simulink model "qdqd_robot"  (R2022b)
settings: Solver=FixedStepAuto  StartTime=0.0  StopTime=10  FixedStep=0.01  RelTol=1e-3  EnableMultiTasking=on
model workspace: external: MATLAB File C:\Users\Tin\Desktop\tailieuhoc\TT Robotics\task2\robot_DataFile2.m (data not in the file)
undefined symbols (not defined in the file): smiData, X, Y, Z
libraries: sm_lib x21, nesl_utility x4, arduinolib x3
settings Model: ExtModeTrigDuration=2  Creator=Tin  LastModifiedBy=Tin
settings OptimizationCC: EnhancedBackFolding=on  PassReuseOutputArgsAs=Individual arguments  ZeroExternalMemoryAtStartup=off  ZeroInternalMemoryAtStartup=off  MaxStackSize=64  OptimizeBlockOrder=speed  DifferentSizesBufferReuse=on  OptimizationCustomize=off  EfficientTunableParamExpr=on
settings DebuggingCC: ParameterTunabilityLossMsg=error
settings HardwareCC: ProdBitPerInt=16  ProdBitPerPointer=16  ProdBitPerSizeT=16  ProdBitPerPtrDiffT=16  ProdLargestAtomicFloat=None  ProdWordSize=8  ProdHWDeviceType=Atmel->AVR
settings SFSimCC: MATLABDynamicMemAlloc=off
settings RTWCC: Description=Embedded Coder  SystemTargetFile=ert.tlc  HardwareBoard=Arduino Uno  TLCOptions=-aInlineSetEventsForThisBaseRateFcn=TLC_FALSE -aSuppressMultiTaskScheduler=TLC_FALSE -aRateBasedStepFcn=1  TemplateMakefile=ert_default_tmf  Toolchain=Arduino AVR  BuildConfiguration=Faster Runs
settings CodeAppCC: ForceParamTrailComments=on  IgnoreCustomStorageClasses=off  OperatorAnnotations=on  SimulinkDataObjDesc=on  SFDataObjDesc=on  InsertBlockDesc=on
settings ERTTargetCC: SupportContinuousTime=on  SupportVariableSizeSignals=on  ExtModeTransport=3  ExtModeStaticAlloc=on  ExtModeAutomaticAllocSize=off  ExtModeStaticAllocSize=250  ExtModeMexFile=ext_xcp  ExtModeIntrfLevel=Level2 - Open

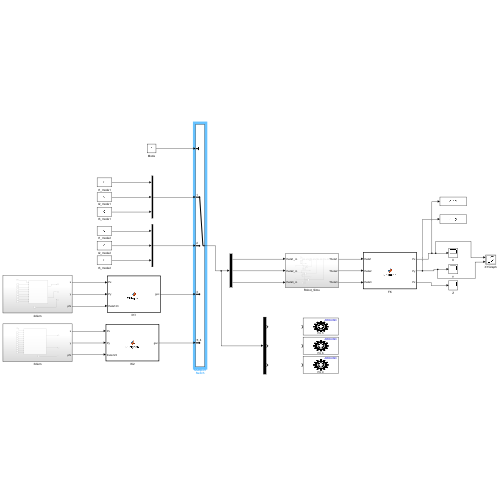
[thumbnail: Simulink's stored preview of the top-level diagram]
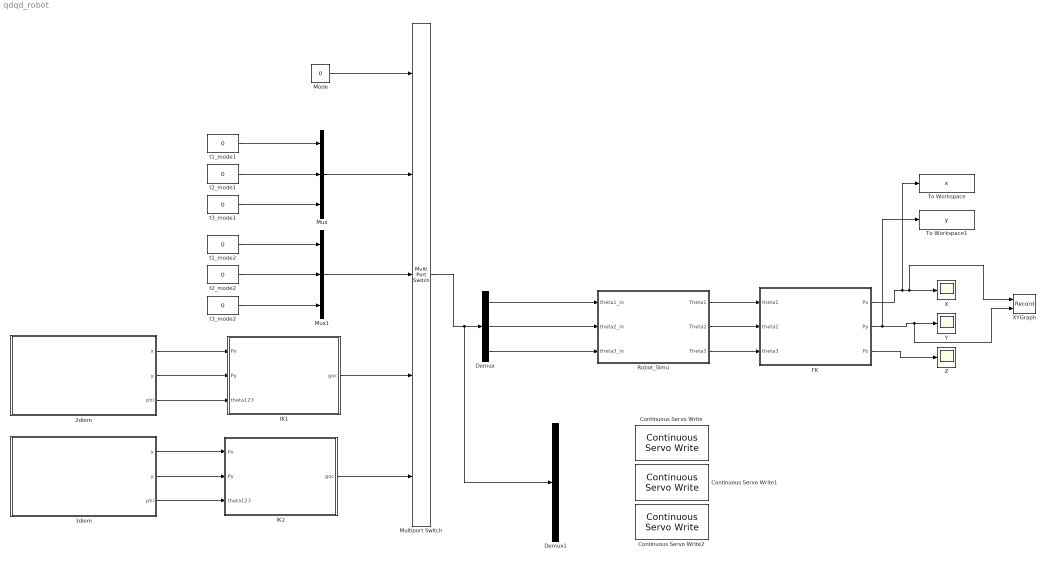
== system qdqd_robot ==
  2diem : Subsystem
  3diem : Subsystem
  Continuous Servo Write : arduinolib/Continuous Servo Write  pinNumber=5  ServoIndex=0  blockPlatform=ARDUINO
  Continuous Servo Write1 : arduinolib/Continuous Servo Write  pinNumber=6  ServoIndex=1  blockPlatform=ARDUINO
  Continuous Servo Write2 : arduinolib/Continuous Servo Write  pinNumber=9  ServoIndex=2  blockPlatform=ARDUINO
  Demux : Demux  Outputs=3
  Demux1 : Demux  Outputs=3
  FK : MATLAB Function  TreatAsAtomicUnit=on
  IK1 : MATLAB Function  TreatAsAtomicUnit=on
  IK2 : MATLAB Function  TreatAsAtomicUnit=on
  Mode : Constant  Value=0
  Multiport Switch : MultiPortSwitch  Inputs=4  DiagnosticForDefault=None  SaturateOnIntegerOverflow=off  InputSameDT=off
  Mux : Mux  Inputs=3
  Mux1 : Mux  Inputs=3
  Robot_Simu : Subsystem
  To Workspace : ToWorkspace  VariableName=x  SampleTime=-1
      settings: Save2DSignal=2-D array (concatenate along first dimension)
  To Workspace1 : ToWorkspace  VariableName=y  SampleTime=-1
      settings: Save2DSignal=2-D array (concatenate along first dimension)
  X : Scope
  XYGraph : Record  FileSettingsInternal="{\"entries\":[{\"content\":{\"excelSettings\":{\"content\":{},\"type\":\"Streamout.ExcelSettings\"}},\"type\":\"Streamout.FileSettingStorage\",\"uuid\":\"e4239a1c-dab3-499a-a52f-9dc0fa17a419\"}],\"packageUris\":[\"http://schema.mathworks.com/mf0/streamout_blocks/R2020a\"],\"version\":\"1.0\"}"  Layout=[1 1]  SignalsInternal="{\"entries\":[{\"content\":{\"signals\":[{\"content\":{\"blockPath\":[\"qdqd_robot/XYGraph\"],\"channel\":[],\"dimensions\":[1],\"domain\":\"qdqd_robot/XYGraph\",\"lineColor\":\"#ff6929\",\"plots\":[],\"port\":1,\"sid\":[\"\"],\"signalID\":171,\"signalName\":\"FK:1\"},\"type\":\"RecordBlkView.Signal\",\"uuid\":\"71b2b6ee-b9d0-4eec-b635-3188d7877590\"},{\"content\":{\"blockPath\":[\"qdqd_robot/XYGraph\"],\"channel\":[],\"dimensions\":[1],\"domain\":\"qdqd_robot/XYGraph\",\"lineColor\":\"#b746ff\",\"plots\":[],\"port\":2,\"sid\":[\"\"],\"signalID\":175,\"signalName\":\"FK:2\"},\"type\":\"RecordBlkView.Signal\",\"uuid\":\"dff031ee-cb77-442e-8ca7-25a6e18e3c29\"}]},\"type\":\"RecordBlkView.InputSignals\",\"uuid\":\"b65a76cf-75d9-49b1-9cf8-3691b3f56b91\"}],\"packageUris\":[\"http://schema.mathworks.com/mf0/streamout_blocks/R2020a\"],\"version\":\"1.0\"}"  VisualizationBindings="{\"xyplotplugin\":{\"info\":[{\"series\":[],\"subplotID\":1}]}}"  CompatibilityTag=XY
  Y : Scope
  Z : Scope
  t1_mode1 : Constant  Value=0
  t1_mode2 : Constant  Value=0
  t2_mode1 : Constant  Value=0
  t2_mode2 : Constant  Value=0
  t3_mode1 : Constant  Value=0
  t3_mode2 : Constant  Value=0
  wires:
  2diem/3(phi) -> IK1/3(theta123)
  2diem/2(y) -> IK1/2(Py)
  3diem/3(phi) -> IK2/3(theta123)
  t2_mode1/1 -> Mux/2
  t3_mode1/1 -> Mux/3
  Mux/1 -> Multiport Switch/2
  Demux/2 -> Robot_Simu/2(theta2_in)
  Demux/3 -> Robot_Simu/3(theta3_in)
  Multiport Switch/1 -> Demux1/1, Demux/1
  t1_mode1/1 -> Mux/1
  3diem/2(y) -> IK2/2(Py)
  3diem/1(x) -> IK2/1(Px)
  Robot_Simu/1(Theta1) -> FK/1(theta1)
  Robot_Simu/2(Theta2) -> FK/2(theta2)
  Robot_Simu/3(Theta3) -> FK/3(theta3)
  FK/1(Px) -> To Workspace/1, XYGraph/1, X/1
  FK/2(Py) -> To Workspace1/1, XYGraph/2, Y/1
  FK/3(Pz) -> Z/1
  Demux/1 -> Robot_Simu/1(theta1_in)
  2diem/1(x) -> IK1/1(Px)
  Mode/1 -> Multiport Switch/1
  IK2/1(goc) -> Multiport Switch/5
  IK1/1(goc) -> Multiport Switch/4
  t1_mode2/1 -> Mux1/1
  Mux1/1 -> Multiport Switch/3
  t3_mode2/1 -> Mux1/3
  t2_mode2/1 -> Mux1/2

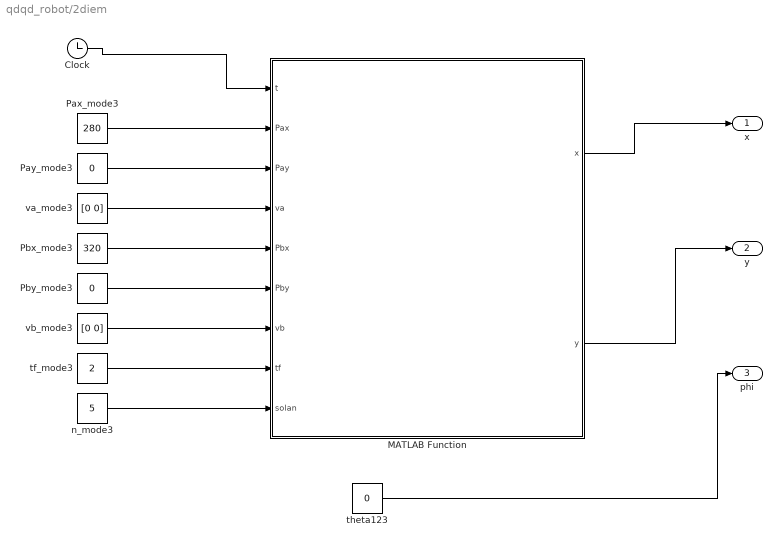
== system qdqd_robot/2diem ==
  Clock : Clock
  MATLAB Function : MATLAB Function  TreatAsAtomicUnit=on
  Pax_mode3 : Constant  Value=280
  Pay_mode3 : Constant  Value=0
  Pbx_mode3 : Constant  Value=320
  Pby_mode3 : Constant  Value=0
  n_mode3 : Constant  Value=5
  tf_mode3 : Constant  Value=2
  theta123 : Constant  Value=0
  va_mode3 : Constant  Value=[0 0]
  vb_mode3 : Constant  Value=[0 0]
  x : Outport
  y : Outport  Port=2
  phi : Outport  Port=3
  wires:
  Pbx_mode3/1 -> MATLAB Function/5(Pbx)
  Pax_mode3/1 -> MATLAB Function/2(Pax)
  Pby_mode3/1 -> MATLAB Function/6(Pby)
  Clock/1 -> MATLAB Function/1(t)
  tf_mode3/1 -> MATLAB Function/8(tf)
  n_mode3/1 -> MATLAB Function/9(solan)
  vb_mode3/1 -> MATLAB Function/7(vb)
  va_mode3/1 -> MATLAB Function/4(va)
  Pay_mode3/1 -> MATLAB Function/3(Pay)
  MATLAB Function/1(x) -> x/1
  theta123/1 -> phi/1
  MATLAB Function/2(y) -> y/1

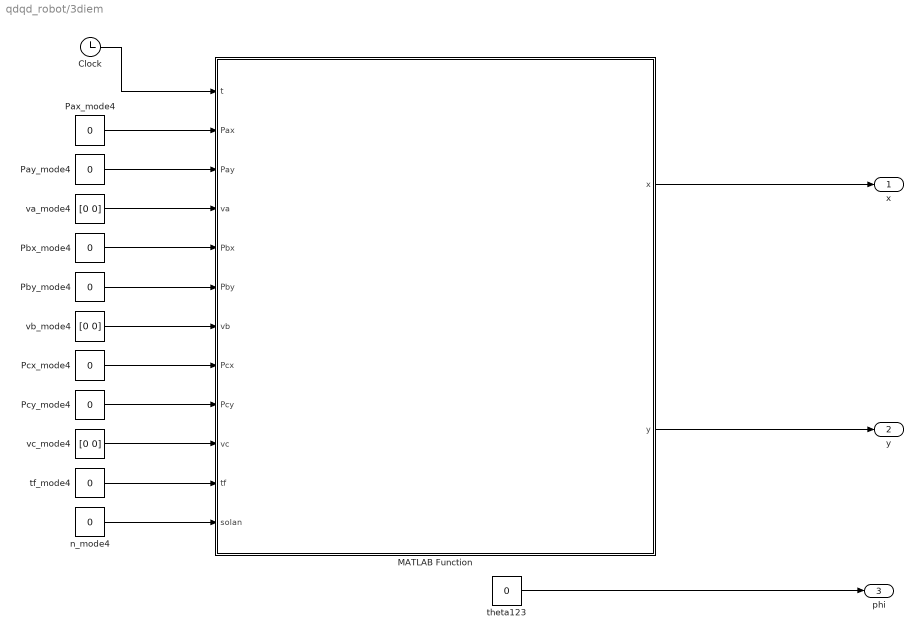
== system qdqd_robot/3diem ==
  Clock : Clock
      settings: Decimation=30
  MATLAB Function : MATLAB Function  TreatAsAtomicUnit=on
  Pax_mode4 : Constant  Value=0
  Pay_mode4 : Constant  Value=0
  Pbx_mode4 : Constant  Value=0
  Pby_mode4 : Constant  Value=0
  Pcx_mode4 : Constant  Value=0
  Pcy_mode4 : Constant  Value=0
  n_mode4 : Constant  Value=0
  tf_mode4 : Constant  Value=0
  theta123 : Constant  Value=0
  va_mode4 : Constant  Value=[0 0]
  vb_mode4 : Constant  Value=[0 0]
  vc_mode4 : Constant  Value=[0 0]
  x : Outport
  y : Outport  Port=2
  phi : Outport  Port=3
  wires:
  theta123/1 -> phi/1
  Pcx_mode4/1 -> MATLAB Function/8(Pcx)
  Pcy_mode4/1 -> MATLAB Function/9(Pcy)
  Pbx_mode4/1 -> MATLAB Function/5(Pbx)
  vc_mode4/1 -> MATLAB Function/10(vc)
  tf_mode4/1 -> MATLAB Function/11(tf)
  Pax_mode4/1 -> MATLAB Function/2(Pax)
  va_mode4/1 -> MATLAB Function/4(va)
  Clock/1 -> MATLAB Function/1(t)
  Pby_mode4/1 -> MATLAB Function/6(Pby)
  Pay_mode4/1 -> MATLAB Function/3(Pay)
  vb_mode4/1 -> MATLAB Function/7(vb)
  n_mode4/1 -> MATLAB Function/12(solan)
  MATLAB Function/1(x) -> x/1
  MATLAB Function/2(y) -> y/1

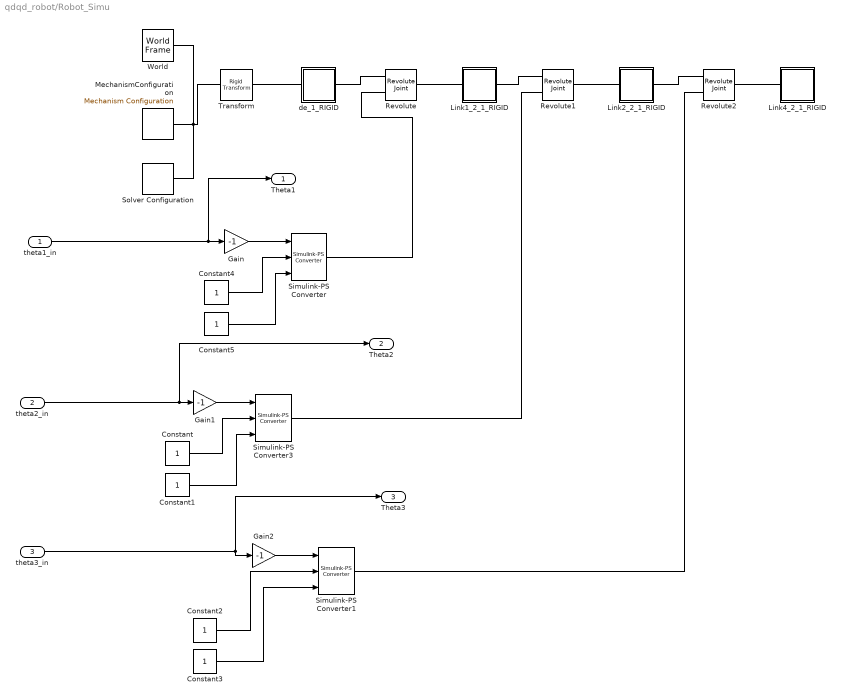
== system qdqd_robot/Robot_Simu ==
  theta1_in : Inport
  theta2_in : Inport  Port=2
  theta3_in : Inport  Port=3
  Constant{,1..5} (6 alike) : Constant
  Gain : Gain  Gain=-1
  Gain1 : Gain  Gain=-1
  Gain2 : Gain  Gain=-1
  Link1_2_1_RIGID : Subsystem
  Link2_2_1_RIGID : Subsystem
  Link4_2_1_RIGID : Subsystem
  MechanismConfiguration : sm_lib/Utilities/Mechanism Configuration  UniformGravity=Constant  GravityVector=[0 -9.80665 0]  GravityUnits=m/s^2  LinearizationDelta=0.001  JointModeTransitionNonlinearIterations=2
  Revolute : sm_lib/Joints/Revolute Joint  JointMode=Normal  SenseConstraintForce=off  SenseConstraintForceX=off  SenseConstraintForceY=off  SenseConstraintForceZ=off  SenseConstraintTorque=off  SenseConstraintTorqueX=off  SenseConstraintTorqueY=off  SenseConstraintTorqueZ=off  SenseTotalForce=off  SenseTotalForceX=off  SenseTotalForceY=off  SenseTotalForceZ=off  SenseTotalTorque=off  SenseTotalTorqueX=off  SenseTotalTorqueY=off  SenseTotalTorqueZ=off  CompositeWrenchDir=FollowerOnBase  CompositeWrenchFrame=BaseFrame  EquilibriumPosition=0  EquilibriumPositionUnits=deg  SpringStiffness=0  SpringStiffnessUnits=N*m/deg  DampingCoefficient=0  DampingCoefficientUnits=N*m/(deg/s)  TorqueActuationMode=ComputedTorque  MotionActuationMode=InputMotion  SensePosition=off  SenseVelocity=off  SenseAcceleration=off  SenseTorqueForce=off  SenseLowerLimitTorqueForce=off  SenseUpperLimitTorqueForce=off  LowerLimitSpecify=off  LowerLimitBound=-90  LowerLimitBoundUnits=deg  LowerLimitStiffness=1e4  LowerLimitStiffnessUnits=N*m/deg  LowerLimitDamping=10  LowerLimitDampingUnits=N*m/(deg/s)  LowerLimitTransitionRegionWidth=0.1  LowerLimitTransitionRegionWidthUnits=deg  UpperLimitSpecify=off  UpperLimitBound=90  UpperLimitBoundUnits=deg  UpperLimitStiffness=1e4  UpperLimitStiffnessUnits=N*m/deg  UpperLimitDamping=10  UpperLimitDampingUnits=N*m/(deg/s)  UpperLimitTransitionRegionWidth=0.1  UpperLimitTransitionRegionWidthUnits=deg  PositionTargetSpecify=on  PositionTargetPriority=Low  PositionTargetValue=smiData.RevoluteJoint(1).Rz.Pos  PositionTargetValueUnits=deg  VelocityTargetSpecify=off  VelocityTargetPriority=High  VelocityTargetValue=0  VelocityTargetValueUnits=deg/s
  Revolute1 : sm_lib/Joints/Revolute Joint  JointMode=Normal  SenseConstraintForce=off  SenseConstraintForceX=off  SenseConstraintForceY=off  SenseConstraintForceZ=off  SenseConstraintTorque=off  SenseConstraintTorqueX=off  SenseConstraintTorqueY=off  SenseConstraintTorqueZ=off  SenseTotalForce=off  SenseTotalForceX=off  SenseTotalForceY=off  SenseTotalForceZ=off  SenseTotalTorque=off  SenseTotalTorqueX=off  SenseTotalTorqueY=off  SenseTotalTorqueZ=off  CompositeWrenchDir=FollowerOnBase  CompositeWrenchFrame=BaseFrame  EquilibriumPosition=0  EquilibriumPositionUnits=deg  SpringStiffness=0  SpringStiffnessUnits=N*m/deg  DampingCoefficient=0  DampingCoefficientUnits=N*m/(deg/s)  TorqueActuationMode=ComputedTorque  MotionActuationMode=InputMotion  SensePosition=off  SenseVelocity=off  SenseAcceleration=off  SenseTorqueForce=off  SenseLowerLimitTorqueForce=off  SenseUpperLimitTorqueForce=off  LowerLimitSpecify=off  LowerLimitBound=-90  LowerLimitBoundUnits=deg  LowerLimitStiffness=1e4  LowerLimitStiffnessUnits=N*m/deg  LowerLimitDamping=10  LowerLimitDampingUnits=N*m/(deg/s)  LowerLimitTransitionRegionWidth=0.1  LowerLimitTransitionRegionWidthUnits=deg  UpperLimitSpecify=off  UpperLimitBound=90  UpperLimitBoundUnits=deg  UpperLimitStiffness=1e4  UpperLimitStiffnessUnits=N*m/deg  UpperLimitDamping=10  UpperLimitDampingUnits=N*m/(deg/s)  UpperLimitTransitionRegionWidth=0.1  UpperLimitTransitionRegionWidthUnits=deg  PositionTargetSpecify=on  PositionTargetPriority=Low  PositionTargetValue=smiData.RevoluteJoint(2).Rz.Pos  PositionTargetValueUnits=deg  VelocityTargetSpecify=off  VelocityTargetPriority=High  VelocityTargetValue=0  VelocityTargetValueUnits=deg/s
  Revolute2 : sm_lib/Joints/Revolute Joint  JointMode=Normal  SenseConstraintForce=off  SenseConstraintForceX=off  SenseConstraintForceY=off  SenseConstraintForceZ=off  SenseConstraintTorque=off  SenseConstraintTorqueX=off  SenseConstraintTorqueY=off  SenseConstraintTorqueZ=off  SenseTotalForce=off  SenseTotalForceX=off  SenseTotalForceY=off  SenseTotalForceZ=off  SenseTotalTorque=off  SenseTotalTorqueX=off  SenseTotalTorqueY=off  SenseTotalTorqueZ=off  CompositeWrenchDir=FollowerOnBase  CompositeWrenchFrame=BaseFrame  EquilibriumPosition=0  EquilibriumPositionUnits=deg  SpringStiffness=0  SpringStiffnessUnits=N*m/deg  DampingCoefficient=0  DampingCoefficientUnits=N*m/(deg/s)  TorqueActuationMode=ComputedTorque  MotionActuationMode=InputMotion  SensePosition=off  SenseVelocity=off  SenseAcceleration=off  SenseTorqueForce=off  SenseLowerLimitTorqueForce=off  SenseUpperLimitTorqueForce=off  LowerLimitSpecify=off  LowerLimitBound=-90  LowerLimitBoundUnits=deg  LowerLimitStiffness=1e4  LowerLimitStiffnessUnits=N*m/deg  LowerLimitDamping=10  LowerLimitDampingUnits=N*m/(deg/s)  LowerLimitTransitionRegionWidth=0.1  LowerLimitTransitionRegionWidthUnits=deg  UpperLimitSpecify=off  UpperLimitBound=90  UpperLimitBoundUnits=deg  UpperLimitStiffness=1e4  UpperLimitStiffnessUnits=N*m/deg  UpperLimitDamping=10  UpperLimitDampingUnits=N*m/(deg/s)  UpperLimitTransitionRegionWidth=0.1  UpperLimitTransitionRegionWidthUnits=deg  PositionTargetSpecify=on  PositionTargetPriority=Low  PositionTargetValue=smiData.RevoluteJoint(3).Rz.Pos  PositionTargetValueUnits=deg  VelocityTargetSpecify=off  VelocityTargetPriority=High  VelocityTargetValue=0  VelocityTargetValueUnits=deg/s
  Simulink-PS Converter : nesl_utility/Simulink-PS Converter  PhysicalDomain=network_engine_domain  SubClassName=ps_input  LeftPortType=input  RightPortType=output  PseudoPeriodic=off  Frequencies=[]  NoiseDistribution=none  NoiseParameters=[]  Unit=1  AffineConversion=on  FilteringAndDerivatives=provide  SimscapeFilterOrder=2  InputFilterTimeConstant=0.001  UdotUserProvided=2
  Simulink-PS Converter1 : nesl_utility/Simulink-PS Converter  PhysicalDomain=network_engine_domain  SubClassName=ps_input  LeftPortType=input  RightPortType=output  PseudoPeriodic=off  Frequencies=[]  NoiseDistribution=none  NoiseParameters=[]  Unit=1  AffineConversion=on  FilteringAndDerivatives=provide  SimscapeFilterOrder=2  InputFilterTimeConstant=0.001  UdotUserProvided=2
  Simulink-PS Converter3 : nesl_utility/Simulink-PS Converter  PhysicalDomain=network_engine_domain  SubClassName=ps_input  LeftPortType=input  RightPortType=output  PseudoPeriodic=off  Frequencies=[]  NoiseDistribution=none  NoiseParameters=[]  Unit=1  AffineConversion=on  FilteringAndDerivatives=provide  SimscapeFilterOrder=2  InputFilterTimeConstant=0.001  UdotUserProvided=2
  Solver Configuration : nesl_utility/Solver Configuration  PhysicalDomain=network_engine_domain  SubClassName=solver  LeftPortType=input  RightPortType=generic  Tones=[]  Harmonics=[]  SimulateNoise=off  Profile=off  UseLocalSampling=off  EnableSwitchedLinearOptims=on  FrequencyDomain=off  UseCCode=off  RelTol=0.001  AbsTol=0.001  MinStep=1e-09  ToWorkspace=off  RevertToSquareIcSolve=off  NumHomotopyIterations=100  PhasorMode=off  PhasorModeNumHarmonics=1  ConsistencySolver=NEWTON_XTOL_AFTER_FTOL  IndexReductionMethod=DerivativeReplacement  DoDC=off  ResidualTolerance=1e-09  ConsistencyTolSource=GLOBAL  ConsistencyAbsTol=0.001  ConsistencyRelTol=0.001  ConsistencyTolFactor=0.001  UseLocalSolver=off  LocalSolverChoice=NE_BACKWARD_EULER_ADVANCER  ResolveIndetEquations=on  FunctionEvalNumThread=1  LocalSolverSampleTime=0.001  DoFixedCost=off  MaxNonlinIter=3  MaxModeIter=2  ComputeImpulses=off  ImpulseIterations=2  LinearAlgebra=auto  LinearAlgebraNumThread=0  EquationFormulation=NE_TIME_EF  DelaysMemoryBudget=1024  AutomaticFiltering=on  FilteringTimeConstant=0.001  PartitionStorageMethod=AS_NEEDED  PartitionMemoryBudget=1024  PartitionMethod=ROBUST
  Transform : sm_lib/Frames and Transforms/Rigid Transform  TranslationMethod=Cartesian  TranslationStandardOffset=0  TranslationLengthUnit=mm  TranslationStandardAxis=+Z  TranslationCartesianOffset=smiData.RigidTransform(2).translation  TranslationROffset=0  TranslationROffsetUnits=m  TranslationZOffset=0  TranslationZOffsetUnits=m  TranslationThetaOffset=0  TranslationThetaOffsetUnits=deg  RotationMethod=ArbitraryAxis  RotationAngleUnits=rad  RotationStandardAxis=+Z  RotationAngle=smiData.RigidTransform(2).angle  RotationArbitraryAxis=smiData.RigidTransform(2).axis  FollAlignAxisA=+X  BaseAlignAxisA=+Y  FollAlignAxisB=+Y  BaseAlignAxisB=+Z  RotationSequenceAxes=FollowerAxes  RotationSequence=XYX  RotationSequenceAngles=[0 0 0]  RotationSequenceAnglesUnits=deg  RotationMatrix=[1 0 0; 0 1 0; 0 0 1]  Quaternion=[1 0 0 0]
  World : sm_lib/Frames and Transforms/World Frame
  de_1_RIGID : Subsystem
  Theta1 : Outport
  Theta2 : Outport  Port=2
  Theta3 : Outport  Port=3
  wires:
  theta2_in/1 -> Theta2/1, Gain1/1
  Gain1/1 -> Simulink-PS Converter3/1
  Gain2/1 -> Simulink-PS Converter1/1
  Constant/1 -> Simulink-PS Converter3/2
  Constant1/1 -> Simulink-PS Converter3/3
  Constant2/1 -> Simulink-PS Converter1/2
  Constant3/1 -> Simulink-PS Converter1/3
  Constant4/1 -> Simulink-PS Converter/2
  Constant5/1 -> Simulink-PS Converter/3
  Gain/1 -> Simulink-PS Converter/1
  theta1_in/1 -> Theta1/1, Gain/1
  theta3_in/1 -> Gain2/1, Theta3/1
  connections:
  World/RConn1 -- MechanismConfiguration/RConn1 -- Solver Configuration/RConn1 -- Transform/LConn1
  Simulink-PS Converter/RConn1 -- Revolute/LConn2
  Link1_2_1_RIGID/LConn1 -- Revolute/RConn1
  Link2_2_1_RIGID/RConn1 -- Revolute2/LConn1
  Transform/RConn1 -- de_1_RIGID/LConn1
  Link2_2_1_RIGID/LConn1 -- Revolute1/RConn1
  Link4_2_1_RIGID/LConn1 -- Revolute2/RConn1
  Revolute/LConn1 -- de_1_RIGID/RConn1
  Link1_2_1_RIGID/RConn1 -- Revolute1/LConn1
  Revolute1/LConn2 -- Simulink-PS Converter3/RConn1
  Simulink-PS Converter1/RConn1 -- Revolute2/LConn2

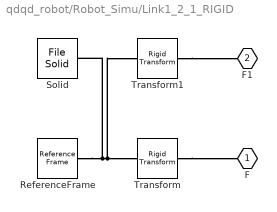
== system qdqd_robot/Robot_Simu/Link1_2_1_RIGID ==
  ReferenceFrame : sm_lib/Frames and Transforms/Reference Frame
  Solid : sm_lib/Body Elements/File Solid  ExtGeomFileName=C:\Users\Tin\Desktop\tailieuhoc\TT Robotics\task2\Link1_2_Default_sldprt.STEP  UnitType=FromFile  ExtGeomFileUnits=m  StepReaderType=HEX  ExportConvexHullGeometry=off  InertiaType=Custom  Mass=smiData.Solid(3).mass  MassUnits=kg  CenterOfMass=smiData.Solid(3).CoM  CenterOfMassUnits=mm  MomentsOfInertia=smiData.Solid(3).MoI  MomentsOfInertiaUnits=kg*mm^2  ProductsOfInertia=smiData.Solid(3).PoI  ProductsOfInertiaUnits=kg*mm^2  BasedOnType=DensityFromFile  Density=1000  DensityUnits=kg/m^3  DoExposeReferenceFrame=on  SerializedFrames=<Frames/>  GraphicType=FromGeometry  MarkerShape=Sphere  MarkerSize=10  GraphicVisPropType=SimpleVisualProperties  GraphicDiffuseColor=smiData.Solid(3).color  GraphicSpecularColor=[0.5 0.5 0.5 1.0]  GraphicAmbientColor=[0.15 0.15 0.15 1.0]  GraphicEmissiveColor=[0.0 0.0 0.0 1.0]  GraphicShininess=75  GraphicOpacity=smiData.Solid(3).opacity
  Transform : sm_lib/Frames and Transforms/Rigid Transform  TranslationMethod=Cartesian  TranslationStandardOffset=0  TranslationLengthUnit=mm  TranslationStandardAxis=+Z  TranslationCartesianOffset=smiData.RigidTransform(4).translation  TranslationROffset=0  TranslationROffsetUnits=m  TranslationZOffset=0  TranslationZOffsetUnits=m  TranslationThetaOffset=0  TranslationThetaOffsetUnits=deg  RotationMethod=ArbitraryAxis  RotationAngleUnits=rad  RotationStandardAxis=+Z  RotationAngle=smiData.RigidTransform(4).angle  RotationArbitraryAxis=smiData.RigidTransform(4).axis  FollAlignAxisA=+X  BaseAlignAxisA=+Y  FollAlignAxisB=+Y  BaseAlignAxisB=+Z  RotationSequenceAxes=FollowerAxes  RotationSequence=XYX  RotationSequenceAngles=[0 0 0]  RotationSequenceAnglesUnits=deg  RotationMatrix=[1 0 0; 0 1 0; 0 0 1]  Quaternion=[1 0 0 0]
  Transform1 : sm_lib/Frames and Transforms/Rigid Transform  TranslationMethod=Cartesian  TranslationStandardOffset=0  TranslationLengthUnit=mm  TranslationStandardAxis=+Z  TranslationCartesianOffset=smiData.RigidTransform(5).translation  TranslationROffset=0  TranslationROffsetUnits=m  TranslationZOffset=0  TranslationZOffsetUnits=m  TranslationThetaOffset=0  TranslationThetaOffsetUnits=deg  RotationMethod=ArbitraryAxis  RotationAngleUnits=rad  RotationStandardAxis=+Z  RotationAngle=smiData.RigidTransform(5).angle  RotationArbitraryAxis=smiData.RigidTransform(5).axis  FollAlignAxisA=+X  BaseAlignAxisA=+Y  FollAlignAxisB=+Y  BaseAlignAxisB=+Z  RotationSequenceAxes=FollowerAxes  RotationSequence=XYX  RotationSequenceAngles=[0 0 0]  RotationSequenceAnglesUnits=deg  RotationMatrix=[1 0 0; 0 1 0; 0 0 1]  Quaternion=[1 0 0 0]
  F : PMIOPort  Side=Left
  F1 : PMIOPort  Port=2  Side=Right
  connections:
  ReferenceFrame/RConn1 -- Transform/LConn1 -- Transform1/LConn1 -- Solid/RConn1
  Transform/RConn1 -- F/RConn1
  Transform1/RConn1 -- F1/RConn1

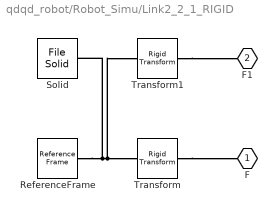
== system qdqd_robot/Robot_Simu/Link2_2_1_RIGID ==
  ReferenceFrame : sm_lib/Frames and Transforms/Reference Frame
  Solid : sm_lib/Body Elements/File Solid  ExtGeomFileName=C:\Users\Tin\Desktop\tailieuhoc\TT Robotics\task2\Link2_2_Default_sldprt.STEP  UnitType=FromFile  ExtGeomFileUnits=m  StepReaderType=HEX  ExportConvexHullGeometry=off  InertiaType=Custom  Mass=smiData.Solid(4).mass  MassUnits=kg  CenterOfMass=smiData.Solid(4).CoM  CenterOfMassUnits=mm  MomentsOfInertia=smiData.Solid(4).MoI  MomentsOfInertiaUnits=kg*mm^2  ProductsOfInertia=smiData.Solid(4).PoI  ProductsOfInertiaUnits=kg*mm^2  BasedOnType=DensityFromFile  Density=1000  DensityUnits=kg/m^3  DoExposeReferenceFrame=on  SerializedFrames=<Frames/>  GraphicType=FromGeometry  MarkerShape=Sphere  MarkerSize=10  GraphicVisPropType=SimpleVisualProperties  GraphicDiffuseColor=smiData.Solid(4).color  GraphicSpecularColor=[0.5 0.5 0.5 1.0]  GraphicAmbientColor=[0.15 0.15 0.15 1.0]  GraphicEmissiveColor=[0.0 0.0 0.0 1.0]  GraphicShininess=75  GraphicOpacity=smiData.Solid(4).opacity
  Transform : sm_lib/Frames and Transforms/Rigid Transform  TranslationMethod=Cartesian  TranslationStandardOffset=0  TranslationLengthUnit=mm  TranslationStandardAxis=+Z  TranslationCartesianOffset=smiData.RigidTransform(6).translation  TranslationROffset=0  TranslationROffsetUnits=m  TranslationZOffset=0  TranslationZOffsetUnits=m  TranslationThetaOffset=0  TranslationThetaOffsetUnits=deg  RotationMethod=ArbitraryAxis  RotationAngleUnits=rad  RotationStandardAxis=+Z  RotationAngle=smiData.RigidTransform(6).angle  RotationArbitraryAxis=smiData.RigidTransform(6).axis  FollAlignAxisA=+X  BaseAlignAxisA=+Y  FollAlignAxisB=+Y  BaseAlignAxisB=+Z  RotationSequenceAxes=FollowerAxes  RotationSequence=XYX  RotationSequenceAngles=[0 0 0]  RotationSequenceAnglesUnits=deg  RotationMatrix=[1 0 0; 0 1 0; 0 0 1]  Quaternion=[1 0 0 0]
  Transform1 : sm_lib/Frames and Transforms/Rigid Transform  TranslationMethod=Cartesian  TranslationStandardOffset=0  TranslationLengthUnit=mm  TranslationStandardAxis=+Z  TranslationCartesianOffset=smiData.RigidTransform(7).translation  TranslationROffset=0  TranslationROffsetUnits=m  TranslationZOffset=0  TranslationZOffsetUnits=m  TranslationThetaOffset=0  TranslationThetaOffsetUnits=deg  RotationMethod=ArbitraryAxis  RotationAngleUnits=rad  RotationStandardAxis=+Z  RotationAngle=smiData.RigidTransform(7).angle  RotationArbitraryAxis=smiData.RigidTransform(7).axis  FollAlignAxisA=+X  BaseAlignAxisA=+Y  FollAlignAxisB=+Y  BaseAlignAxisB=+Z  RotationSequenceAxes=FollowerAxes  RotationSequence=XYX  RotationSequenceAngles=[0 0 0]  RotationSequenceAnglesUnits=deg  RotationMatrix=[1 0 0; 0 1 0; 0 0 1]  Quaternion=[1 0 0 0]
  F : PMIOPort  Side=Left
  F1 : PMIOPort  Port=2  Side=Right
  connections:
  ReferenceFrame/RConn1 -- Transform/LConn1 -- Transform1/LConn1 -- Solid/RConn1
  Transform/RConn1 -- F/RConn1
  Transform1/RConn1 -- F1/RConn1

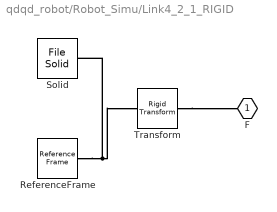
== system qdqd_robot/Robot_Simu/Link4_2_1_RIGID ==
  ReferenceFrame : sm_lib/Frames and Transforms/Reference Frame
  Solid : sm_lib/Body Elements/File Solid  ExtGeomFileName=C:\Users\Tin\Desktop\tailieuhoc\TT Robotics\task2\Link4_2_Default_sldprt.STEP  UnitType=FromFile  ExtGeomFileUnits=m  StepReaderType=HEX  ExportConvexHullGeometry=off  InertiaType=Custom  Mass=smiData.Solid(1).mass  MassUnits=kg  CenterOfMass=smiData.Solid(1).CoM  CenterOfMassUnits=mm  MomentsOfInertia=smiData.Solid(1).MoI  MomentsOfInertiaUnits=kg*mm^2  ProductsOfInertia=smiData.Solid(1).PoI  ProductsOfInertiaUnits=kg*mm^2  BasedOnType=DensityFromFile  Density=1000  DensityUnits=kg/m^3  DoExposeReferenceFrame=on  SerializedFrames=<Frames/>  GraphicType=FromGeometry  MarkerShape=Sphere  MarkerSize=10  GraphicVisPropType=SimpleVisualProperties  GraphicDiffuseColor=smiData.Solid(1).color  GraphicSpecularColor=[0.5 0.5 0.5 1.0]  GraphicAmbientColor=[0.15 0.15 0.15 1.0]  GraphicEmissiveColor=[0.0 0.0 0.0 1.0]  GraphicShininess=75  GraphicOpacity=smiData.Solid(1).opacity
  Transform : sm_lib/Frames and Transforms/Rigid Transform  TranslationMethod=Cartesian  TranslationStandardOffset=0  TranslationLengthUnit=mm  TranslationStandardAxis=+Z  TranslationCartesianOffset=smiData.RigidTransform(8).translation  TranslationROffset=0  TranslationROffsetUnits=m  TranslationZOffset=0  TranslationZOffsetUnits=m  TranslationThetaOffset=0  TranslationThetaOffsetUnits=deg  RotationMethod=ArbitraryAxis  RotationAngleUnits=rad  RotationStandardAxis=+Z  RotationAngle=smiData.RigidTransform(8).angle  RotationArbitraryAxis=smiData.RigidTransform(8).axis  FollAlignAxisA=+X  BaseAlignAxisA=+Y  FollAlignAxisB=+Y  BaseAlignAxisB=+Z  RotationSequenceAxes=FollowerAxes  RotationSequence=XYX  RotationSequenceAngles=[0 0 0]  RotationSequenceAnglesUnits=deg  RotationMatrix=[1 0 0; 0 1 0; 0 0 1]  Quaternion=[1 0 0 0]
  F : PMIOPort  Side=Left
  connections:
  ReferenceFrame/RConn1 -- Solid/RConn1 -- Transform/LConn1
  Transform/RConn1 -- F/RConn1

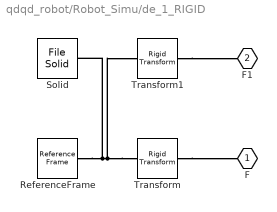
== system qdqd_robot/Robot_Simu/de_1_RIGID ==
  ReferenceFrame : sm_lib/Frames and Transforms/Reference Frame
  Solid : sm_lib/Body Elements/File Solid  ExtGeomFileName=C:\Users\Tin\Desktop\tailieuhoc\TT Robotics\task2\de_Default_sldprt.STEP  UnitType=FromFile  ExtGeomFileUnits=m  StepReaderType=HEX  ExportConvexHullGeometry=off  InertiaType=Custom  Mass=smiData.Solid(2).mass  MassUnits=kg  CenterOfMass=smiData.Solid(2).CoM  CenterOfMassUnits=mm  MomentsOfInertia=smiData.Solid(2).MoI  MomentsOfInertiaUnits=kg*mm^2  ProductsOfInertia=smiData.Solid(2).PoI  ProductsOfInertiaUnits=kg*mm^2  BasedOnType=DensityFromFile  Density=1000  DensityUnits=kg/m^3  DoExposeReferenceFrame=on  SerializedFrames=<Frames/>  GraphicType=FromGeometry  MarkerShape=Sphere  MarkerSize=10  GraphicVisPropType=SimpleVisualProperties  GraphicDiffuseColor=smiData.Solid(2).color  GraphicSpecularColor=[0.5 0.5 0.5 1.0]  GraphicAmbientColor=[0.15 0.15 0.15 1.0]  GraphicEmissiveColor=[0.0 0.0 0.0 1.0]  GraphicShininess=75  GraphicOpacity=smiData.Solid(2).opacity
  Transform : sm_lib/Frames and Transforms/Rigid Transform  TranslationMethod=Cartesian  TranslationStandardOffset=0  TranslationLengthUnit=mm  TranslationStandardAxis=+Z  TranslationCartesianOffset=smiData.RigidTransform(1).translation  TranslationROffset=0  TranslationROffsetUnits=m  TranslationZOffset=0  TranslationZOffsetUnits=m  TranslationThetaOffset=0  TranslationThetaOffsetUnits=deg  RotationMethod=ArbitraryAxis  RotationAngleUnits=rad  RotationStandardAxis=+Z  RotationAngle=smiData.RigidTransform(1).angle  RotationArbitraryAxis=smiData.RigidTransform(1).axis  FollAlignAxisA=+X  BaseAlignAxisA=+Y  FollAlignAxisB=+Y  BaseAlignAxisB=+Z  RotationSequenceAxes=FollowerAxes  RotationSequence=XYX  RotationSequenceAngles=[0 0 0]  RotationSequenceAnglesUnits=deg  RotationMatrix=[1 0 0; 0 1 0; 0 0 1]  Quaternion=[1 0 0 0]
  Transform1 : sm_lib/Frames and Transforms/Rigid Transform  TranslationMethod=Cartesian  TranslationStandardOffset=0  TranslationLengthUnit=mm  TranslationStandardAxis=+Z  TranslationCartesianOffset=smiData.RigidTransform(3).translation  TranslationROffset=0  TranslationROffsetUnits=m  TranslationZOffset=0  TranslationZOffsetUnits=m  TranslationThetaOffset=0  TranslationThetaOffsetUnits=deg  RotationMethod=ArbitraryAxis  RotationAngleUnits=rad  RotationStandardAxis=+Z  RotationAngle=smiData.RigidTransform(3).angle  RotationArbitraryAxis=smiData.RigidTransform(3).axis  FollAlignAxisA=+X  BaseAlignAxisA=+Y  FollAlignAxisB=+Y  BaseAlignAxisB=+Z  RotationSequenceAxes=FollowerAxes  RotationSequence=XYX  RotationSequenceAngles=[0 0 0]  RotationSequenceAnglesUnits=deg  RotationMatrix=[1 0 0; 0 1 0; 0 0 1]  Quaternion=[1 0 0 0]
  F : PMIOPort  Side=Left
  F1 : PMIOPort  Port=2  Side=Right
  connections:
  Transform/LConn1 -- Transform1/LConn1 -- ReferenceFrame/RConn1 -- Solid/RConn1
  Transform/RConn1 -- F/RConn1
  Transform1/RConn1 -- F1/RConn1

== matlab function qdqd_robot/IK1 ==
  data: Px input; goc output; Py input; theta123 input
function goc  = DHNghich(Px, Py, theta123)
    l1 = 100;
    l2 = 250;
    l3 = 250;
    l4 = 150;
    %tinh theta2
    nx = Px - l1 -l4*cosd(theta123);
    ny = Py - l4*sind(theta123);

    s2 = sqrt(complex(1 - ((nx^2 + ny^2 - l2^2 - l3^2) / (2 * l2 * l3))^2));
    s2 = real(s2);
    c2 = (nx^2 + ny^2 - l2^2 - l3^2) / (2 * l2 * l3);
    theta2 = atan2d (s2, c2);

    %tinh theta1
    A1 = ny * (l2 + l3 * cosd(theta2)) - l3*sind(theta2)*nx;
    A2 = (l2 + l3*cosd(theta2))^2 + (l3*sind(theta2))^2;
    A = A1/A2;

    B = (nx + l3*sind(theta2)*A) / (l2 + l3*cosd(theta2));
    theta1 = atan2d(A, B);
    %tinh theta3
    theta3 = theta123 - (theta2 + theta1);
    goc = [theta1; theta2; theta3];
end

== matlab function qdqd_robot/2diem/MATLAB Function ==
  data: x output; t input; y output; Pax input; Pay input; va input; Pbx input; Pby input; vb input; tf input; solan input
function [x, y] = QHQD2D(t, Pax, Pay, va, Pbx, Pby, vb, tf, solan)

    function [x, y] = TrajectoryPlanning(t, P0, v0, Pf, vf, tf, t0)
        a10 = P0(1);
        a20 = P0(2);
        a11 = v0(1);
        a21 = v0(2);  
    
        a12 = 3 / tf^2 * (Pf(1) - P0(1)) - 2 / tf * v0(1) - 1 / tf * vf(1);
        a22 = 3 / tf^2 * (Pf(2) - P0(2)) - 2 / tf * v0(2) - 1 / tf * vf(2);
        a13 = -2 / tf^3 * (Pf(1) - P0(1)) + 1 / tf^2 * (vf(1) + v0(1));
        a23 = -2 / tf^3 * (Pf(2) - P0(2)) + 1 / tf^2 * (vf(2) + v0(2));
    
        x = a10 + a11 *(t - t0) + a12 * (t - t0)^2 + a13*(t - t0)^3;
        y = a20 + a21 *(t - t0) + a22 * (t - t0)^2 + a23*(t - t0)^3;
    end

    chuky = tf*2;
    i = fix(t/chuky);
    Pa = [Pax Pay];
    Pb = [Pbx Pby];
    if(t <= (tf + chuky*i))
        [x, y] = TrajectoryPlanning(t, Pa, va, Pb, vb, tf, 0 + chuky * i);
    else
        [x, y] = TrajectoryPlanning(t, Pa, va, Pb, vb, tf, tf + chuky * i);
    end
    if(t > chuky*solan)
         x = Pax;
         y = Pay;
    end
end

== matlab function qdqd_robot/3diem/MATLAB Function ==
  data: x output; t input; y output; Pax input; Pay input; va input; Pbx input; Pby input; vb input; Pcx input; Pcy input; vc input; tf input; solan input
function [x, y] = QHQD3D(t, Pax, Pay, va, Pbx, Pby, vb, Pcx, Pcy, vc, tf, solan) 
    function [x, y, z] = TrajectoryPlanning(t, P0, v0, Pf, vf, tf, t0)
        a10 = P0(1);
        a20 = P0(2);
        a11 = v0(1);
        a21 = v0(2);  
    
        a12 = 3 / tf^2 * (Pf(1) - P0(1)) - 2 / tf * v0(1) - 1 / tf * vf(1);
        a22 = 3 / tf^2 * (Pf(2) - P0(2)) - 2 / tf * v0(2) - 1 / tf * vf(2);
        a13 = -2 / tf^3 * (Pf(1) - P0(1)) + 1 / tf^2 * (vf(1) + v0(1));
        a23 = -2 / tf^3 * (Pf(2) - P0(2)) + 1 / tf^2 * (vf(2) + v0(2));
    
        x = a10 + a11 *(t - t0) + a12 * (t - t0)^2 + a13*(t - t0)^3;
        y = a20 + a21 *(t - t0) + a22 * (t - t0)^2 + a23*(t - t0)^3;
        z = 0;
    end
    chuky = tf*3;
    i = fix(t/chuky);
    Pa = [Pax Pay];
    Pb = [Pbx Pby];
    Pc = [Pcx Pcy];
    if(t <= (tf + chuky*i))
        [x, y] = TrajectoryPlanning(t, Pa, va, Pb, vb, tf, tf*0 + chuky * i);
    elseif(t <= (tf*2 + chuky*i))
        [x, y] = TrajectoryPlanning(t, Pb, vb, Pc, vc, tf, tf*1 + chuky * i);
    else
        [x, y] = TrajectoryPlanning(t, Pc, vc, Pa, va, tf, tf*2 + chuky * i);
    end
    if(t > chuky*solan)
         x = Pax;
         y = Pay;
    end
end

== matlab function qdqd_robot/IK2 ==
  data: Px input; goc output; Py input; theta123 input
function goc  = DHNghich(Px, Py, theta123)
    l1 = 100;
    l2 = 250;
    l3 = 250;
    l4 = 150;
    %tinh theta2
    nx = Px - l1 -l4*cosd(theta123);
    ny = Py - l4*sind(theta123);

    s2 = sqrt(complex(1 - ((nx^2 + ny^2 - l2^2 - l3^2) / (2 * l2 * l3))^2));
    s2 = real(s2);
    c2 = (nx^2 + ny^2 - l2^2 - l3^2) / (2 * l2 * l3);
    theta2 = atan2d (s2, c2);

    %tinh theta1
    A1 = ny * (l2 + l3 * cosd(theta2)) - l3*sind(theta2)*nx;
    A2 = (l2 + l3*cosd(theta2))^2 + (l3*sind(theta2))^2;
    A = A1/A2;

    B = (nx + l3*sind(theta2)*A) / (l2 + l3*cosd(theta2));
    theta1 = atan2d(A, B);
    %tinh theta3
    theta3 = theta123 - (theta2 + theta1);
    goc = [theta1; theta2; theta3];
end

== matlab function qdqd_robot/FK ==
  data: theta1 input; Px output; theta2 input; theta3 input; Py output; Pz output
function [Px, Py, Pz] = DHThuan(theta1, theta2, theta3)
    l1 = 100;
    l2 = 250;
    l3 = 250;
    l4 = 150;
    d1 = 30;
    d2 = 30;
    d3 = 30;
    l0 = 150;

    theta123= 0;

    Px = l1 + l2*cosd(theta1) + l3*cosd(theta1 + theta2) + l4*cosd(theta123);
    Py = l2*sind(theta1) + l3*sind(theta1 + theta2) + l4*sind(theta123);
    Pz = l0 + d1 + d2 + d3;
end
